simulink model "ParamTest"  (R2020a)
settings: Solver=FixedStepAuto  StartTime=0.0  StopTime=10.0  FixedStep=1e-3  RelTol=1e-3  EnableMultiTasking=on
libraries: simulink x2, frdmk64flib x2, etargetslib x1
settings Model: SimulationMode=external  ExtModeTrigDuration=5  Creator=WinnieTrandinh  LastModifiedBy=WinnieTrandinh
settings OptimizationCC: EnhancedBackFolding=on  PassReuseOutputArgsAs=Individual arguments  ZeroExternalMemoryAtStartup=off  ZeroInternalMemoryAtStartup=off  MaxStackSize=64  OptimizeBlockOrder=speed  DifferentSizesBufferReuse=on  OptimizationCustomize=off  EfficientTunableParamExpr=on
settings DebuggingCC: ParameterTunabilityLossMsg=error
settings HardwareCC: ProdBitPerPointer=32  ProdBitPerSizeT=32  ProdBitPerPtrDiffT=32  ProdLargestAtomicInteger=Long  ProdLargestAtomicFloat=Double  ProdWordSize=32  ProdHWDeviceType=ARM Compatible->ARM Cortex
settings SFSimCC: MATLABDynamicMemAlloc=off
settings RTWCC: SystemTargetFile=ert.tlc  HardwareBoard=NXP FRDM-K64F  TemplateMakefile=ert_default_tmf  Toolchain=GNU Tools for ARM Embedded Processors
settings CodeAppCC: ForceParamTrailComments=on  IgnoreCustomStorageClasses=off  OperatorAnnotations=on  SimulinkDataObjDesc=on  SFDataObjDesc=on  InsertBlockDesc=on
settings ERTTargetCC: ExtMode=on  ExtModeTransport=4  ExtModeMexFile=sendToCommService  ExtModeMexArgs='ParamTest' 0

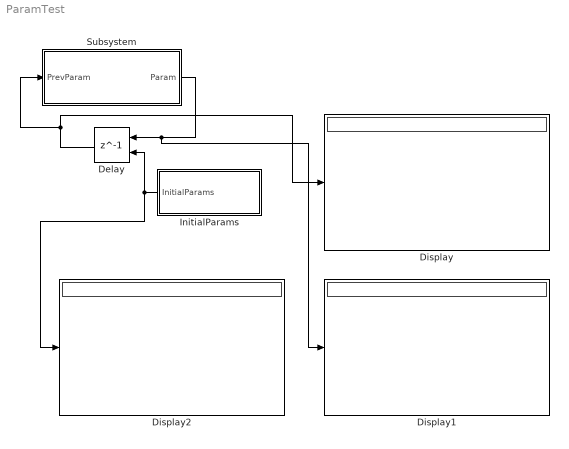
== system ParamTest ==
  Delay : Delay  DelayLength=1  InitialConditionSource=Input port  InitialCondition=[1000 5 10 5 10 300 400 3.5 3.5 500 0.1 16 5000 5000 1 100 1 1 1]
      settings: InputPortMap=u0,p4
  Display : Display
  Display1 : Display
  Display2 : Display
  InitialParams : Subsystem
  Subsystem : Subsystem
  wires:
  InitialParams/1(InitialParams) -> Display2/1, Delay/2
  Subsystem/1(Param) -> Display1/1, Delay/1
  Delay/1 -> Subsystem/1(PrevParam), Display/1

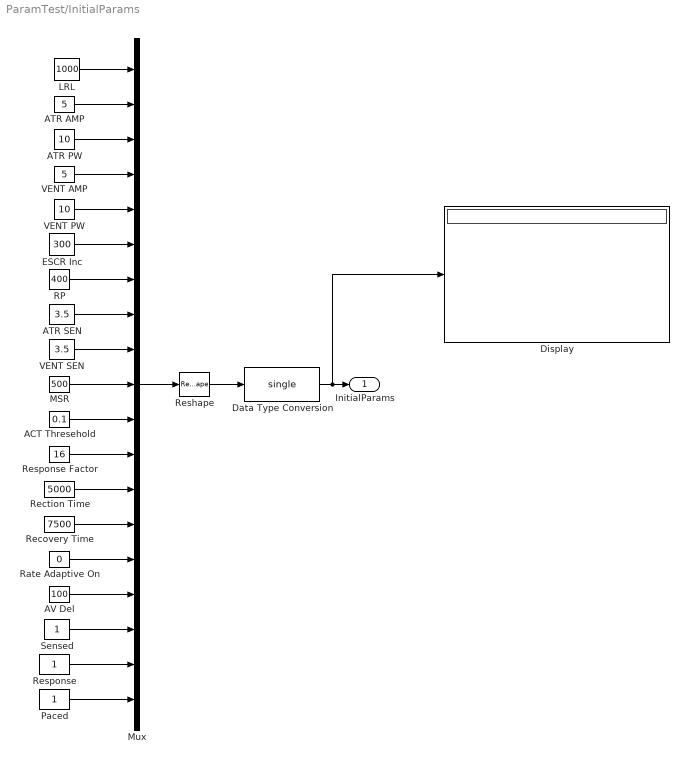
== system ParamTest/InitialParams ==
  " ACT Thresehold" : Constant  Value=0.1
  " MSR" : Constant  Value=500
  " VENT AMP" : Constant  Value=5
  ATR AMP : Constant  Value=5
  ATR PW : Constant  Value=10
  ATR SEN : Constant  Value=3.5
  AV Del : Constant  Value=100
  Data Type Conversion : DataTypeConversion  OutDataTypeStr=single
  Display : Display
  ESCR Inc : Constant  Value=300
  LRL : Constant  Value=1000
  Mux : Mux  Inputs=19
  Paced : Constant
  RP : Constant  Value=400
  Rate Adaptive On : Constant  Value=0
  Recovery Time : Constant  Value=7500
  Rection Time : Constant  Value=5000
  Reshape : Reshape  OutputDimensionality=Row vector (2-D)
  Response : Constant
  Response Factor : Constant  Value=16
  Sensed : Constant
  VENT PW : Constant  Value=10
  VENT SEN : Constant  Value=3.5
  InitialParams : Outport
  wires:
  LRL/1 -> Mux/1
  ATR AMP/1 -> Mux/2
  ATR PW/1 -> Mux/3
  " VENT AMP"/1 -> Mux/4
  VENT PW/1 -> Mux/5
  ESCR Inc/1 -> Mux/6
  RP/1 -> Mux/7
  ATR SEN/1 -> Mux/8
  VENT SEN/1 -> Mux/9
  " MSR"/1 -> Mux/10
  " ACT Thresehold"/1 -> Mux/11
  Response Factor/1 -> Mux/12
  Rection Time/1 -> Mux/13
  Recovery Time/1 -> Mux/14
  Rate Adaptive On/1 -> Mux/15
  AV Del/1 -> Mux/16
  Sensed/1 -> Mux/17
  Response/1 -> Mux/18
  Paced/1 -> Mux/19
  Mux/1 -> Reshape/1
  Reshape/1 -> Data Type Conversion/1
  Data Type Conversion/1 -> Display/1, InitialParams/1

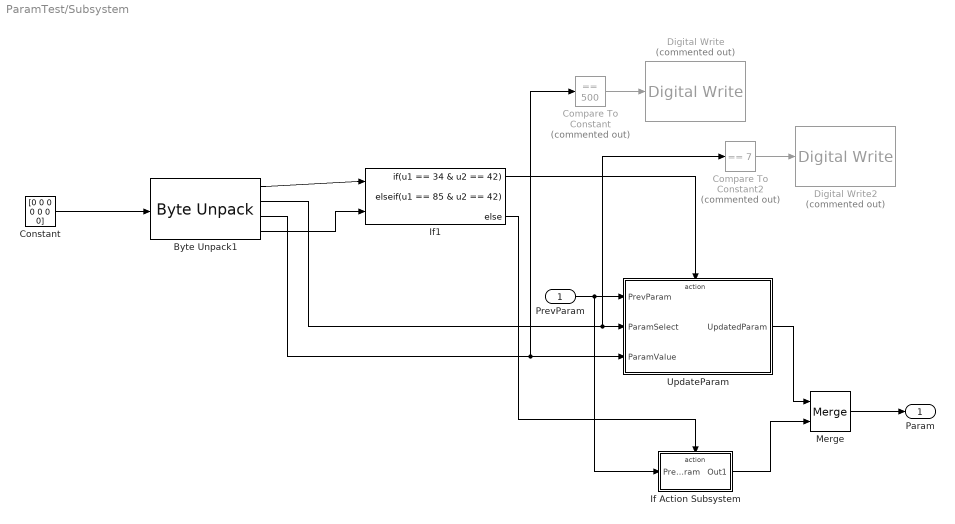
== system ParamTest/Subsystem ==
  PrevParam : Inport
  Byte Unpack1 : etargetslib/Byte Unpack  dimensions={1 1 1 1}  datatypes={'uint8', 'uint8', 'single', 'uint8'}  byteAlign=1
  Compare To Constant : simulink/Logic and Bit Operations/Compare To Constant  Commented=on  relop===  const=500  OutDataTypeStr=boolean
  Compare To Constant2 : simulink/Logic and Bit Operations/Compare To Constant  Commented=on  relop===  const=7  OutDataTypeStr=boolean
  Constant : Constant  Value=[0 0 0 0 0 0 0]  OutDataTypeStr=uint8
  Digital Write : frdmk64flib/Digital Write  Commented=on  Whichpin=GREEN_LED
  Digital Write2 : frdmk64flib/Digital Write  Commented=on  Whichpin=BLUE_LED
  If Action Subsystem : Subsystem  TreatAsAtomicUnit=on
  If1 : If  NumInputs=2  IfExpression=u1 == 34 & u2 == 42  ElseIfExpressions=u1 == 85 & u2 == 42
  Merge : Merge
  UpdateParam : Subsystem
  Param : Outport
  wires:
  Byte Unpack1/3 -> UpdateParam/3(ParamValue), Compare To Constant/1
  If1/1 -> UpdateParam/Action
  Byte Unpack1/4 -> If1/2
  PrevParam/1 -> If Action Subsystem/1(PrevParam), UpdateParam/1(PrevParam)
  Byte Unpack1/2 -> Compare To Constant2/1, UpdateParam/2(ParamSelect)
  Byte Unpack1/1 -> If1/1
  UpdateParam/1(UpdatedParam) -> Merge/1
  Compare To Constant2/1 -> Digital Write2/1
  Constant/1 -> Byte Unpack1/1
  Compare To Constant/1 -> Digital Write/1
  If1/3 -> If Action Subsystem/Action
  If Action Subsystem/1(Out1) -> Merge/2
  Merge/1 -> Param/1

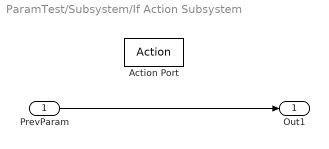
== system ParamTest/Subsystem/If Action Subsystem ==
  PrevParam : Inport
  Action Port : ActionPort  ActionPortLabel=else
  Out1 : Outport
  wires:
  PrevParam/1 -> Out1/1

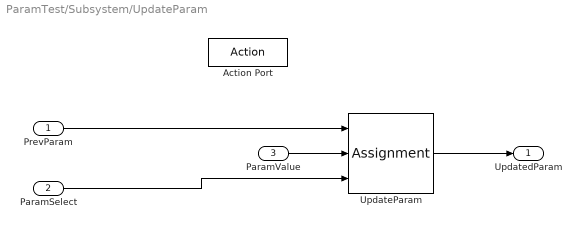
== system ParamTest/Subsystem/UpdateParam ==
  PrevParam : Inport  OutDataTypeStr=single  PortDimensions=[1 19]
  ParamSelect : Inport  Port=2
  ParamValue : Inport  Port=3
  Action Port : ActionPort  ActionPortLabel=if(u1 == 34 & u2 == 42)
  UpdateParam : Assignment  DiagnosticForDimensions=Warning  IndexOptions=Index vector (port)  Indices=1  OutputSizes=1
  UpdatedParam : Outport
  wires:
  PrevParam/1 -> UpdateParam/1
  UpdateParam/1 -> UpdatedParam/1
  ParamSelect/1 -> UpdateParam/3
  ParamValue/1 -> UpdateParam/2
